simulink subsystem "rss_RefElecSpdCalcHybr"  (R2023a)
settings: Solver=VariableStepAuto  StartTime=0.0  StopTime=10.0  RelTol=1e-3
undefined symbols (not defined in the file): Cdbl_nElecAgSpdMaxVal, Cdbl_nElecAgSpdPeakVal, Cdbl_nMechSpdMaxVal, Cdbl_nMechSpdPeakVal, ENM_MOTO_STATUS, Gs16_nAlgnRefElecSpd_C, Gs16_nLmpHmeRefMechSpd_C, Gs16_nMaxStrtUpRefElecSpd_C, Gs16_nMinSenlRefElecSpd_C, Gs16_nUDS2FRefMechSpd_C, Gu16_ctAlgnStEndCnt_C
libraries: simulink x11, lib_configurable_parameter x3, lib_conversion x2, lib_dynamic_saturator x2, vhit_control_library x2, lib_rate_limiter_YXQ x2
settings Model: Creator=xiaoqiang.yuan  LastModifiedBy=xiaoqiang.yuan

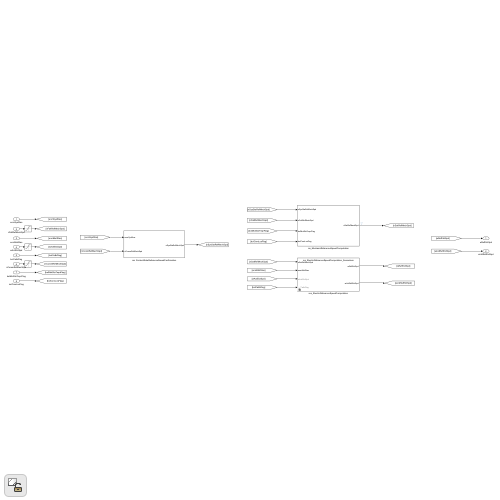
[thumbnail: Simulink's stored preview of the top-level diagram]
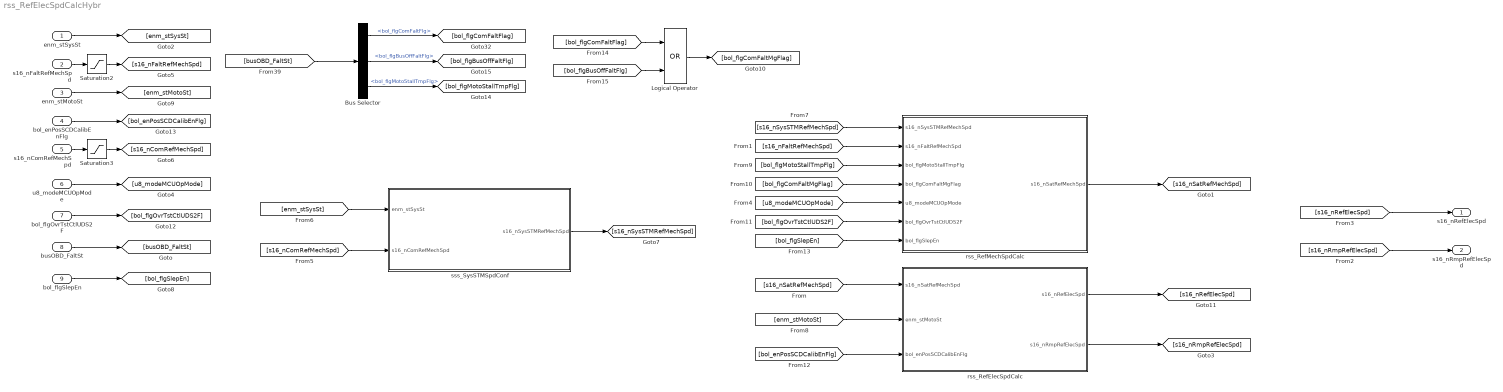
== system rss_RefElecSpdCalcHybr ==
  enm_stSysSt : Inport  OutDataTypeStr=Enum: ENM_SYS_STATUS
  s16_nFaltRefMechSpd : Inport  Port=2  OutDataTypeStr=dt_Standardize_s16p15b0
  enm_stMotoSt : Inport  Port=3  OutDataTypeStr=Enum: ENM_MOTO_STATUS
  bol_enPosSCDCalibEnFlg : Inport  Port=4  OutDataTypeStr=boolean
  s16_nComRefMechSpd : Inport  Port=5  OutDataTypeStr=dt_Standardize_s16p15b0
  u8_modeMCUOpMode : Inport  Port=6  OutDataTypeStr=uint8
  bol_flgOvrTstCtlUDS2F : Inport  Port=7  OutDataTypeStr=boolean
  busOBD_FaltSt : Inport  Port=8  OutDataTypeStr=Bus: BUS_OBD_FALT_STS
  bol_flgSlepEn : Inport  Port=9  OutDataTypeStr=boolean
  Bus Selector : BusSelector  OutputSignals=bol_flgComFaltFlg,bol_flgBusOffFaltFlg,bol_flgMotoStallTmpFlg
  Logical Operator : Logic  Operator=OR  AllPortsSameDT=off  OutDataTypeStr=boolean
  Saturation2 : Saturate  UpperLimit=Cdbl_nMechSpdMaxVal  LowerLimit=-Cdbl_nMechSpdMaxVal
  Saturation3 : Saturate  UpperLimit=Cdbl_nMechSpdMaxVal  LowerLimit=-Cdbl_nMechSpdMaxVal
  rss_RefElecSpdCalc : Subsystem  VariantControl=cstSenlCtrlLbl
  rss_RefMechSpdCalc : Subsystem
  sss_SysSTMSpdConf : Subsystem
  s16_nRefElecSpd : Outport  OutDataTypeStr=dt_Standardize_s16p15b0
  s16_nRmpRefElecSpd : Outport  Port=2  OutDataTypeStr=dt_Standardize_s16p15b0
  wires:
  enm_stMotoSt/1 -> [enm_stMotoSt]
  [s16_nRmpRefElecSpd] -> s16_nRmpRefElecSpd/1
  rss_RefMechSpdCalc/1(s16_nSatRefMechSpd) -> [s16_nSatRefMechSpd]
  [s16_nSysSTMRefMechSpd] -> rss_RefMechSpdCalc/1(s16_nSysSTMRefMechSpd)
  enm_stSysSt/1 -> [enm_stSysSt]
  Saturation2/1 -> [s16_nFaltRefMechSpd]
  s16_nFaltRefMechSpd/1 -> Saturation2/1
  [s16_nFaltRefMechSpd] -> rss_RefMechSpdCalc/2(s16_nFaltRefMechSpd)
  [s16_nRefElecSpd] -> s16_nRefElecSpd/1
  s16_nComRefMechSpd/1 -> Saturation3/1
  Saturation3/1 -> [s16_nComRefMechSpd]
  [s16_nComRefMechSpd] -> sss_SysSTMSpdConf/2(s16_nComRefMechSpd)
  [enm_stSysSt] -> sss_SysSTMSpdConf/1(enm_stSysSt)
  sss_SysSTMSpdConf/1(s16_nSysSTMRefMechSpd) -> [s16_nSysSTMRefMechSpd]
  [bol_flgMotoStallTmpFlg] -> rss_RefMechSpdCalc/3(bol_flgMotoStallTmpFlg)
  [bol_flgComFaltMgFlag] -> rss_RefMechSpdCalc/4(bol_flgComFaltMgFlag)
  rss_RefElecSpdCalc/2(s16_nRmpRefElecSpd) -> [s16_nRmpRefElecSpd]
  rss_RefElecSpdCalc/1(s16_nRefElecSpd) -> [s16_nRefElecSpd]
  [enm_stMotoSt] -> rss_RefElecSpdCalc/2(enm_stMotoSt)
  [s16_nSatRefMechSpd] -> rss_RefElecSpdCalc/1(s16_nSatRefMechSpd)
  u8_modeMCUOpMode/1 -> [u8_modeMCUOpMode]
  [u8_modeMCUOpMode] -> rss_RefMechSpdCalc/5(u8_modeMCUOpMode)
  bol_flgOvrTstCtlUDS2F/1 -> [bol_flgOvrTstCtlUDS2F]
  [bol_flgOvrTstCtlUDS2F] -> rss_RefMechSpdCalc/6(bol_flgOvrTstCtlUDS2F)
  bol_enPosSCDCalibEnFlg/1 -> [bol_enPosSCDCalibEnFlg]
  [bol_enPosSCDCalibEnFlg] -> rss_RefElecSpdCalc/3(bol_enPosSCDCalibEnFlg)
  Bus Selector/1 -> [bol_flgComFaltFlag]  "<bol_flgComFaltFlg>"
  Bus Selector/3 -> [bol_flgMotoStallTmpFlg]  "<bol_flgMotoStallTmpFlg>"
  [busOBD_FaltSt] -> Bus Selector/1
  busOBD_FaltSt/1 -> [busOBD_FaltSt]
  bol_flgSlepEn/1 -> [bol_flgSlepEn]
  [bol_flgSlepEn] -> rss_RefMechSpdCalc/7(bol_flgSlepEn)
  [bol_flgComFaltFlag] -> Logical Operator/1
  [bol_flgBusOffFaltFlg] -> Logical Operator/2
  Logical Operator/1 -> [bol_flgComFaltMgFlag]
  Bus Selector/2 -> [bol_flgBusOffFaltFlg]  "<bol_flgBusOffFaltFlg>"

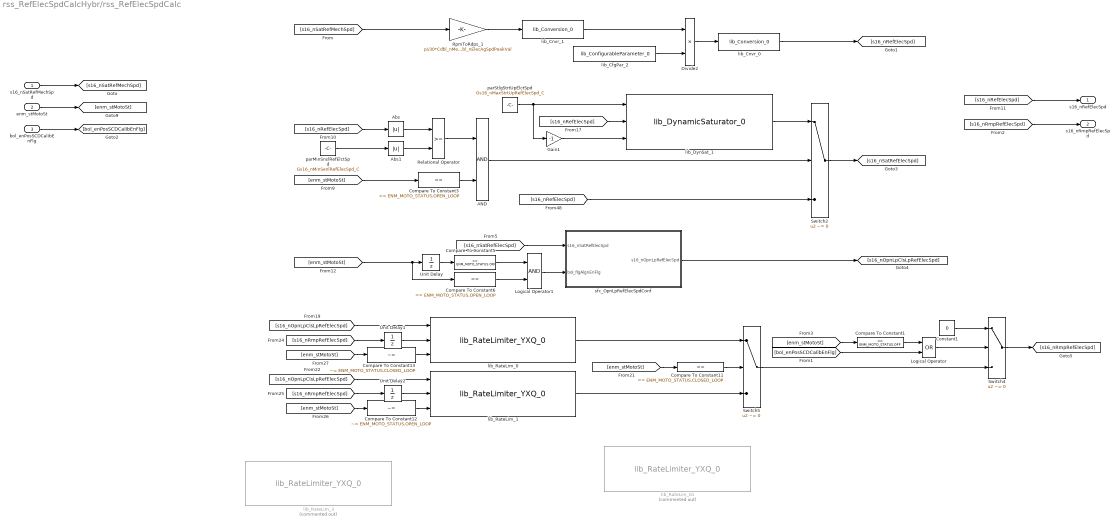
== system rss_RefElecSpdCalcHybr/rss_RefElecSpdCalc ==
  s16_nSatRefMechSpd : Inport
  enm_stMotoSt : Inport  Port=2
  bol_enPosSCDCalibEnFlg : Inport  Port=3
  AND : Logic  AllPortsSameDT=off  OutDataTypeStr=boolean
  Abs : Abs  SaturateOnIntegerOverflow=off
  Abs1 : Abs  SaturateOnIntegerOverflow=off
  Compare To Constant1 : simulink/Logic and Bit Operations/Compare To Constant  relop===  const=ENM_MOTO_STATUS.OFF  OutDataTypeStr=boolean
  Compare To Constant11 : simulink/Logic and Bit Operations/Compare To Constant  relop===  const=ENM_MOTO_STATUS.CLOSED_LOOP  OutDataTypeStr=boolean
  Compare To Constant12 : simulink/Logic and Bit Operations/Compare To Constant  relop=~=  const=ENM_MOTO_STATUS.OPEN_LOOP  OutDataTypeStr=boolean
  Compare To Constant13 : simulink/Logic and Bit Operations/Compare To Constant  relop=~=  const=ENM_MOTO_STATUS.CLOSED_LOOP  OutDataTypeStr=boolean
  Compare To Constant3 : simulink/Logic and Bit Operations/Compare To Constant  relop===  const=ENM_MOTO_STATUS.OPEN_LOOP  OutDataTypeStr=boolean
  Compare To Constant5 : simulink/Logic and Bit Operations/Compare To Constant  relop===  const=ENM_MOTO_STATUS.OFF  OutDataTypeStr=boolean
  Compare To Constant6 : simulink/Logic and Bit Operations/Compare To Constant  relop===  const=ENM_MOTO_STATUS.OPEN_LOOP  OutDataTypeStr=boolean
  Constant1 : Constant  Value=0  OutDataTypeStr=dt_Standardize_s16p15b0
  Divide2 : Product  Inputs=**  OutDataTypeStr=Inherit: Inherit via back propagation  RndMeth=Simplest
  Gain1 : Gain  Gain=-1  OutDataTypeStr=Inherit: Inherit via back propagation
  Logical Operator : Logic  Operator=OR  AllPortsSameDT=off  OutDataTypeStr=boolean
  Logical Operator1 : Logic  AllPortsSameDT=off  OutDataTypeStr=boolean
  Relational Operator : RelationalOperator  OutDataTypeStr=boolean  RndMeth=Simplest  InputSameDT=off
  RpmToRdps_1 : Gain  Gain=pi/30*Cdbl_nMechSpdPeakVal/Cdbl_nElecAgSpdPeakVal  OutDataTypeStr=Inherit: Inherit via back propagation  RndMeth=Simplest
  Switch2 : Switch  Criteria=u2 ~= 0  SaturateOnIntegerOverflow=off  InputSameDT=off
  Switch4 : Switch  Criteria=u2 ~= 0  SaturateOnIntegerOverflow=off  InputSameDT=off
  Switch5 : Switch  Criteria=u2 ~= 0  SaturateOnIntegerOverflow=off  InputSameDT=off
  Unit Delay : UnitDelay  InitialCondition=ENM_MOTO_STATUS.OFF  SampleTime=-1  HasFrameUpgradeWarning=on
  Unit Delay1 : UnitDelay  SampleTime=-1  HasFrameUpgradeWarning=on
  Unit Delay2 : UnitDelay  SampleTime=-1  HasFrameUpgradeWarning=on
  lib_CfgPar_2 : lib_configurable_parameter/lib_ConfigurableParameter_0  lb_parCnfgPar=Gu8_numPPNum_C  lb_parDataType=Inherit: Inherit from 'Constant value'  lb_parUpLim=Cdbl_numPPNumMaxVal  lb_parLowLim=Cdbl_numPPNumMinVal
  lib_Cnvr_0 : lib_conversion/lib_Conversion_0  lb_parDataType=dt_Standardize_s16p15b0  lb_parOutpMaxVal=[]  lb_parOutpMinVal=[]  lb_parSatFlag=off
  lib_Cnvr_1 : lib_conversion/lib_Conversion_0  lb_parDataType=fixdt(1,16)  lb_parOutpMaxVal=pi/30*Cdbl_nMechSpdPeakVal/Cdbl_nElecAgSpdPeakVal  lb_parOutpMinVal=[]  RndMeth=Simplest  lb_parSatFlag=off
  lib_DynSat_1 : lib_dynamic_saturator/lib_DynamicSaturator_0
  lib_RateLim_0 : vhit_control_library/lib_RateLimiter_YXQ_0  lb_parSampTime=Cdbl_tiSlwTaskSmpTi  lb_parRiseSlewRate=Gs16_facRefSpdRisSlwRate_C  lb_parFallSlewRate=Gs16_facRefSpdFallSlwRate_C  lb_parMaxInpVal=Cdbl_nElecAgSpdMaxVal  lb_parMinInpVal=-Cdbl_nElecAgSpdMaxVal
      settings: LibrarySourceBlock=lib_rate_limiter/lib_RateLimiter_0
  lib_RateLim_01 : lib_rate_limiter_YXQ/lib_RateLimiter_YXQ_0  Commented=on  lb_parSampTime=Cdbl_tiSlwTaskSmpTi  lb_parRiseSlewRate=Gs16_facRefSpdRisSlwRate_C  lb_parFallSlewRate=Gs16_facRefSpdFallSlwRate_C  lb_parMaxInpVal=Cdbl_nElecAgSpdMaxVal  lb_parMinInpVal=-Cdbl_nElecAgSpdMaxVal
      settings: LibrarySourceBlock=lib_rate_limiter/lib_RateLimiter_0
  lib_RateLim_1 : vhit_control_library/lib_RateLimiter_YXQ_0  lb_parSampTime=Cdbl_tiSlwTaskSmpTi  lb_parRiseSlewRate=Gs16_facRefSpdOLRiseSlwRate_C  lb_parFallSlewRate=Gs16_facRefSpdOLFallSlwRate_C  lb_parMaxInpVal=Cdbl_nElecAgSpdMaxVal  lb_parMinInpVal=-Cdbl_nElecAgSpdMaxVal
      settings: LibrarySourceBlock=lib_rate_limiter/lib_RateLimiter_0
  lib_RateLim_3 : lib_rate_limiter_YXQ/lib_RateLimiter_YXQ_0  Commented=on  lb_parSampTime=Cdbl_tiSlwTaskSmpTi  lb_parRiseSlewRate=Gs16_facRefSpdOpnLpRiseSlwRate_C  lb_parFallSlewRate=Gs16_facRefSpdOpnLpFallSlwRate_C  lb_parMaxInpVal=Cdbl_nElecAgSpdMaxVal  lb_parMinInpVal=-Cdbl_nElecAgSpdMaxVal
      settings: LibrarySourceBlock=lib_rate_limiter/lib_RateLimiter_0
  parMinSnslRefElctSpd : Constant  Value=Gs16_nMinSenlRefElecSpd_C
  parStlgStrtUpElctSpd : Constant  Value=Gs16_nMaxStrtUpRefElecSpd_C
  sfc_OpnLpRefElecSpdConf : Stateflow chart  TreatAsAtomicUnit=on
  s16_nRefElecSpd : Outport
  s16_nRmpRefElecSpd : Outport  Port=2
  wires:
  bol_enPosSCDCalibEnFlg/1 -> [bol_enPosSCDCalibEnFlg]
  Compare To Constant1/1 -> Logical Operator/1
  [enm_stMotoSt] -> Compare To Constant1/1
  [bol_enPosSCDCalibEnFlg] -> Logical Operator/2
  lib_CfgPar_2/1 -> Divide2/2
  Divide2/1 -> lib_Cnvr_0/1
  lib_Cnvr_1/1 -> Divide2/1
  RpmToRdps_1/1 -> lib_Cnvr_1/1
  lib_Cnvr_0/1 -> [s16_nRefElecSpd]
  [s16_nSatRefMechSpd] -> RpmToRdps_1/1
  Unit Delay2/1 -> lib_RateLim_1/2
  Unit Delay1/1 -> lib_RateLim_0/2
  Compare To Constant13/1 -> lib_RateLim_0/3
  [enm_stMotoSt] -> Compare To Constant13/1
  Compare To Constant12/1 -> lib_RateLim_1/3
  [enm_stMotoSt] -> Compare To Constant12/1
  [s16_nRmpRefElecSpd] -> Unit Delay2/1
  [s16_nRmpRefElecSpd] -> Unit Delay1/1
  lib_RateLim_1/1 -> Switch5/3
  [s16_nOpnLpClsLpRefElecSpd] -> lib_RateLim_1/1
  lib_RateLim_0/1 -> Switch5/1
  Switch4/1 -> [s16_nRmpRefElecSpd]
  Compare To Constant11/1 -> Switch5/2
  [enm_stMotoSt] -> Compare To Constant11/1
  Switch5/1 -> Switch4/3
  Constant1/1 -> Switch4/1
  Logical Operator/1 -> Switch4/2
  [s16_nOpnLpClsLpRefElecSpd] -> lib_RateLim_0/1
  sfc_OpnLpRefElecSpdConf/1(s16_nOpnLpRefElecSpd) -> [s16_nOpnLpClsLpRefElecSpd]
  [s16_nRefElecSpd] -> lib_DynSat_1/2
  Gain1/1 -> lib_DynSat_1/3
  lib_DynSat_1/1 -> Switch2/1
  parStlgStrtUpElctSpd/1 -> Gain1/1, lib_DynSat_1/1
  [s16_nRefElecSpd] -> Switch2/3
  Logical Operator1/1 -> sfc_OpnLpRefElecSpdConf/2(bol_flgAlgnEnFlg)
  [enm_stMotoSt] -> Unit Delay/1, Compare To Constant6/1
  Compare To Constant6/1 -> Logical Operator1/2
  Compare To Constant5/1 -> Logical Operator1/1
  Unit Delay/1 -> Compare To Constant5/1
  [s16_nSatRefElecSpd] -> sfc_OpnLpRefElecSpdConf/1(s16_nSatRefElecSpd)
  [s16_nRefElecSpd] -> s16_nRefElecSpd/1
  [enm_stMotoSt] -> Compare To Constant3/1
  AND/1 -> Switch2/2
  Compare To Constant3/1 -> AND/2
  Abs/1 -> Relational Operator/1
  parMinSnslRefElctSpd/1 -> Abs1/1
  [s16_nRefElecSpd] -> Abs/1
  Abs1/1 -> Relational Operator/2
  Switch2/1 -> [s16_nSatRefElecSpd]
  Relational Operator/1 -> AND/1
  enm_stMotoSt/1 -> [enm_stMotoSt]
  [s16_nRmpRefElecSpd] -> s16_nRmpRefElecSpd/1
  s16_nSatRefMechSpd/1 -> [s16_nSatRefMechSpd]

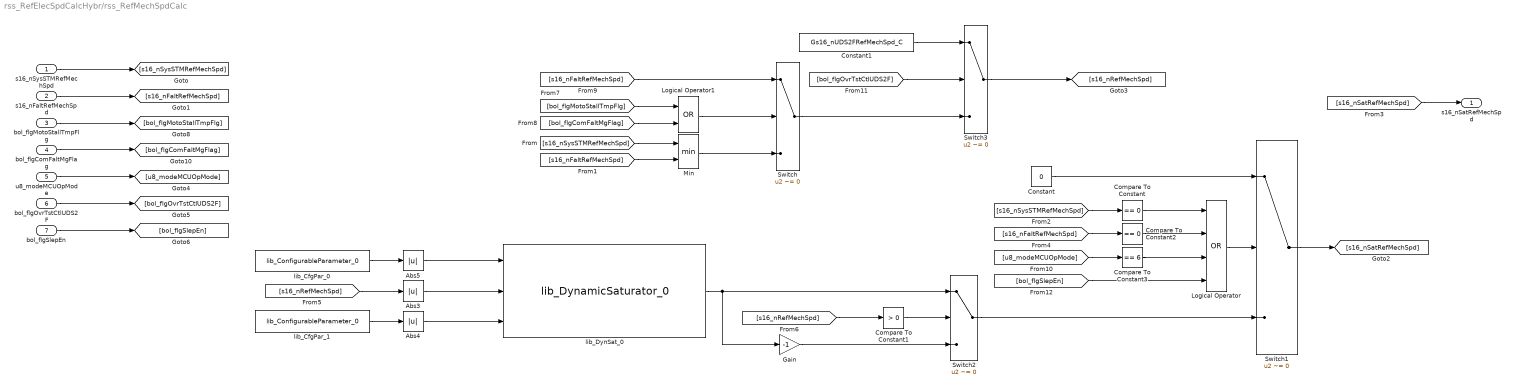
== system rss_RefElecSpdCalcHybr/rss_RefMechSpdCalc ==
  s16_nSysSTMRefMechSpd : Inport
  s16_nFaltRefMechSpd : Inport  Port=2
  bol_flgMotoStallTmpFlg : Inport  Port=3
  bol_flgComFaltMgFlag : Inport  Port=4
  u8_modeMCUOpMode : Inport  Port=5
  bol_flgOvrTstCtlUDS2F : Inport  Port=6
  bol_flgSlepEn : Inport  Port=7
  Abs3 : Abs  SaturateOnIntegerOverflow=off
  Abs4 : Abs  SaturateOnIntegerOverflow=off
  Abs5 : Abs  SaturateOnIntegerOverflow=off
  Compare To Constant : simulink/Logic and Bit Operations/Compare To Constant  relop===  const=0  OutDataTypeStr=boolean
  Compare To Constant1 : simulink/Logic and Bit Operations/Compare To Constant  relop=>  const=0  OutDataTypeStr=boolean
  Compare To Constant2 : simulink/Logic and Bit Operations/Compare To Constant  relop===  const=0  OutDataTypeStr=boolean
  Compare To Constant3 : simulink/Logic and Bit Operations/Compare To Constant  relop===  const=6  OutDataTypeStr=boolean
  Constant : Constant  Value=0  OutDataTypeStr=dt_Standardize_s16p15b0
  Constant1 : Constant  Value=Gs16_nUDS2FRefMechSpd_C
  Gain : Gain  Gain=-1  OutDataTypeStr=Inherit: Same as input
  Logical Operator : Logic  Operator=OR  Inputs=4  AllPortsSameDT=off  OutDataTypeStr=boolean
  Logical Operator1 : Logic  Operator=OR  AllPortsSameDT=off  OutDataTypeStr=boolean
  Min : MinMax  Inputs=2  OutDataTypeStr=Inherit: Same as first input
  Switch{,1..3} (4 alike) : Switch  Criteria=u2 ~= 0  SaturateOnIntegerOverflow=off  InputSameDT=off
  lib_CfgPar_0 : lib_configurable_parameter/lib_ConfigurableParameter_0  lb_parCnfgPar=Gs16_nMaxRefMechSpd_C  lb_parDataType=Inherit: Inherit from 'Constant value'  lb_parUpLim=Cdbl_nMechSpdMaxVal  lb_parLowLim=-Cdbl_nMechSpdMaxVal
  lib_CfgPar_1 : lib_configurable_parameter/lib_ConfigurableParameter_0  lb_parCnfgPar=Gs16_nMinRefMechSpd_C  lb_parDataType=Inherit: Inherit from 'Constant value'  lb_parUpLim=Cdbl_nMechSpdMaxVal  lb_parLowLim=-Cdbl_nMechSpdMaxVal
  lib_DynSat_0 : lib_dynamic_saturator/lib_DynamicSaturator_0
  s16_nSatRefMechSpd : Outport
  wires:
  bol_flgSlepEn/1 -> [bol_flgSlepEn]
  [bol_flgSlepEn] -> Logical Operator/4
  Compare To Constant3/1 -> Logical Operator/3
  bol_flgOvrTstCtlUDS2F/1 -> [bol_flgOvrTstCtlUDS2F]
  Constant1/1 -> Switch3/1
  Switch/1 -> Switch3/3
  Switch3/1 -> [s16_nRefMechSpd]
  [bol_flgOvrTstCtlUDS2F] -> Switch3/2
  [u8_modeMCUOpMode] -> Compare To Constant3/1
  u8_modeMCUOpMode/1 -> [u8_modeMCUOpMode]
  Min/1 -> Switch/3
  [s16_nFaltRefMechSpd] -> Switch/1
  Logical Operator1/1 -> Switch/2
  [bol_flgComFaltMgFlag] -> Logical Operator1/2
  [bol_flgMotoStallTmpFlg] -> Logical Operator1/1
  bol_flgComFaltMgFlag/1 -> [bol_flgComFaltMgFlag]
  bol_flgMotoStallTmpFlg/1 -> [bol_flgMotoStallTmpFlg]
  Switch1/1 -> [s16_nSatRefMechSpd]
  Switch2/1 -> Switch1/3
  lib_DynSat_0/1 -> Switch2/1, Gain/1
  Constant/1 -> Switch1/1
  Logical Operator/1 -> Switch1/2
  [s16_nFaltRefMechSpd] -> Compare To Constant2/1
  [s16_nSysSTMRefMechSpd] -> Compare To Constant/1
  Compare To Constant2/1 -> Logical Operator/2
  Compare To Constant/1 -> Logical Operator/1
  [s16_nFaltRefMechSpd] -> Min/2
  [s16_nSysSTMRefMechSpd] -> Min/1
  s16_nFaltRefMechSpd/1 -> [s16_nFaltRefMechSpd]
  lib_CfgPar_1/1 -> Abs4/1
  [s16_nRefMechSpd] -> Abs3/1
  s16_nSysSTMRefMechSpd/1 -> [s16_nSysSTMRefMechSpd]
  Abs4/1 -> lib_DynSat_0/3
  Abs3/1 -> lib_DynSat_0/2
  [s16_nRefMechSpd] -> Compare To Constant1/1
  [s16_nSatRefMechSpd] -> s16_nSatRefMechSpd/1
  lib_CfgPar_0/1 -> Abs5/1
  Compare To Constant1/1 -> Switch2/2
  Gain/1 -> Switch2/3
  Abs5/1 -> lib_DynSat_0/1

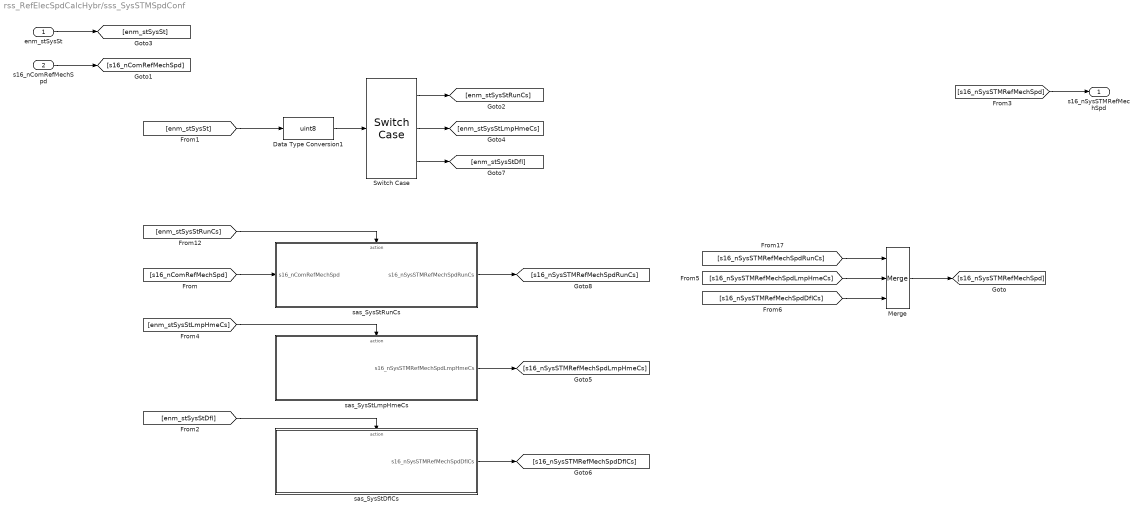
== system rss_RefElecSpdCalcHybr/sss_SysSTMSpdConf ==
  enm_stSysSt : Inport
  s16_nComRefMechSpd : Inport  Port=2
  Data Type Conversion1 : DataTypeConversion  OutDataTypeStr=uint8  SaturateOnIntegerOverflow=off  RndMeth=Floor
  Merge : Merge  Inputs=3
  Switch Case : SwitchCase  CaseConditions={1,5}
  sas_SysStDflCs : Subsystem  TreatAsAtomicUnit=on
  sas_SysStLmpHmeCs : Subsystem  TreatAsAtomicUnit=on
  sas_SysStRunCs : Subsystem  TreatAsAtomicUnit=on
  s16_nSysSTMRefMechSpd : Outport
  wires:
  Data Type Conversion1/1 -> Switch Case/1
  [s16_nSysSTMRefMechSpdDflCs] -> Merge/3
  [s16_nSysSTMRefMechSpdLmpHmeCs] -> Merge/2
  sas_SysStDflCs/1(s16_nSysSTMRefMechSpdDflCs) -> [s16_nSysSTMRefMechSpdDflCs]
  [enm_stSysStDfl] -> sas_SysStDflCs/Action
  [enm_stSysStLmpHmeCs] -> sas_SysStLmpHmeCs/Action
  sas_SysStLmpHmeCs/1(s16_nSysSTMRefMechSpdLmpHmeCs) -> [s16_nSysSTMRefMechSpdLmpHmeCs]
  [enm_stSysSt] -> Data Type Conversion1/1
  enm_stSysSt/1 -> [enm_stSysSt]
  s16_nComRefMechSpd/1 -> [s16_nComRefMechSpd]
  [s16_nSysSTMRefMechSpd] -> s16_nSysSTMRefMechSpd/1
  Switch Case/2 -> [enm_stSysStLmpHmeCs]
  [enm_stSysStRunCs] -> sas_SysStRunCs/Action
  Merge/1 -> [s16_nSysSTMRefMechSpd]
  Switch Case/3 -> [enm_stSysStDfl]
  sas_SysStRunCs/1(s16_nSysSTMRefMechSpdRunCs) -> [s16_nSysSTMRefMechSpdRunCs]
  Switch Case/1 -> [enm_stSysStRunCs]
  [s16_nComRefMechSpd] -> sas_SysStRunCs/1(s16_nComRefMechSpd)
  [s16_nSysSTMRefMechSpdRunCs] -> Merge/1

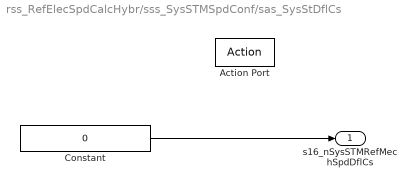
== system rss_RefElecSpdCalcHybr/sss_SysSTMSpdConf/sas_SysStDflCs ==
  Action Port : ActionPort
  Constant : Constant  Value=0  OutDataTypeStr=dt_Standardize_s16p15b0
  s16_nSysSTMRefMechSpdDflCs : Outport
  wires:
  Constant/1 -> s16_nSysSTMRefMechSpdDflCs/1

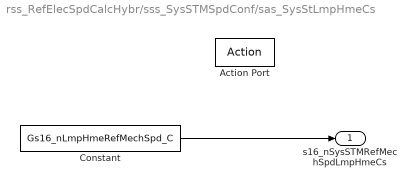
== system rss_RefElecSpdCalcHybr/sss_SysSTMSpdConf/sas_SysStLmpHmeCs ==
  Action Port : ActionPort
  Constant : Constant  Value=Gs16_nLmpHmeRefMechSpd_C
  s16_nSysSTMRefMechSpdLmpHmeCs : Outport
  wires:
  Constant/1 -> s16_nSysSTMRefMechSpdLmpHmeCs/1

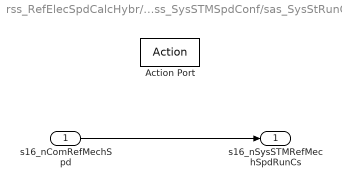
== system rss_RefElecSpdCalcHybr/sss_SysSTMSpdConf/sas_SysStRunCs ==
  s16_nComRefMechSpd : Inport
  Action Port : ActionPort
  s16_nSysSTMRefMechSpdRunCs : Outport
  wires:
  s16_nComRefMechSpd/1 -> s16_nSysSTMRefMechSpdRunCs/1

== stateflow chart rss_RefElecSpdCalcHybr/rss_RefElecSpdCalc/sfc_OpnLpRefElecSpdConf ==
  state STRTUP_SPD
    du:
    s16_nOpnLpRefElecSpd = s16_nSatRefElecSpd;
  state ALGN_SPD
    en:
    s16_nOpnLpRefElecSpd = Gs16_nAlgnRefElecSpd_C;
    u16_ctAlgnStEndCnt = uint16(0);
    du:
    u16_ctAlgnStEndCnt = u16_ctAlgnStEndCnt + uint16(1);
    ex:
    u16_ctAlgnStEndCnt = uint16(0);
  (default) -> STRTUP_SPD
  ALGN_SPD -> STRTUP_SPD : [u16_ctAlgnStEndCnt>= Gu16_ctAlgnStEndCnt_C]
  STRTUP_SPD -> ALGN_SPD : [bol_flgAlgnEnFlg]
  data: s16_nSatRefElecSpd input dt_Standardize_s16p15b0; bol_flgAlgnEnFlg input boolean; u16_ctAlgnStEndCnt local uint16; Gu16_ctAlgnStEndCnt_C parameter; Gs16_nAlgnRefElecSpd_C parameter; s16_nOpnLpRefElecSpd output dt_Standardize_s16p15b0
